simulink model "sideslip_hold"  (R2017a)
settings: Solver=FixedStepAuto  StartTime=0.0  StopTime=10  FixedStep=.001  RelTol=1e-3
values from neighbouring files (symbols this model uses):
  a_beta1 = -P.rho*Va*P.S_wing/(2*P.mass)*P.C_Y_beta    [computeRollGains.m]    (also in compute_gains.m)
  a_beta2 = P.rho*Va*P.S_wing/(2*P.mass)*P.C_Y_delta_r    [computeRollGains.m]    (also in compute_gains.m)
  delta_r_max = 45*pi/180    (= 0.785398163397)    [computeRollGains.m]    (also in compute_gains.m)
  ki_beta = 1/a_beta2*((a_beta1 + a_beta2*kp_beta)/2/zeta_beta)^2    [computeRollGains.m]
  kp_beta = delta_r_max/e_beta_max*sign(a_beta2)    [computeRollGains.m]
settings Model: Creator=pizzaslayer  LastModifiedBy=pizzaslayer

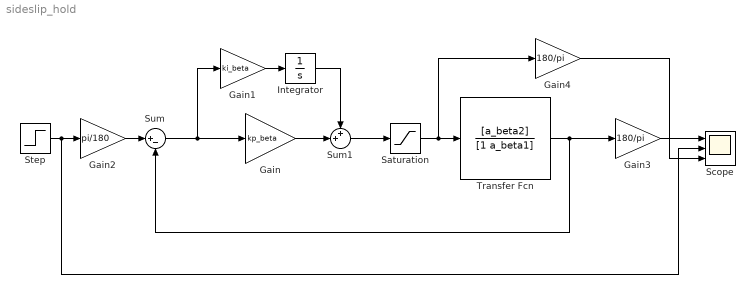
== system sideslip_hold ==
  Gain : Gain  Gain=kp_beta
  Gain1 : Gain  Gain=ki_beta
  Gain2 : Gain  Gain=pi/180
  Gain3 : Gain  Gain=180/pi
  Gain4 : Gain  Gain=180/pi
  Integrator : Integrator  InitialCondition=10*pi/180
  Saturation : Saturate  UpperLimit=delta_r_max  LowerLimit=-delta_r_max
  Scope : Scope  NumInputPorts=3
  Step : Step  Time=2  After=0  SampleTime=0
  Sum : Sum  Inputs=|+-
  Sum1 : Sum  Inputs=++|
  Transfer Fcn : TransferFcn  Numerator=[a_beta2]  Denominator=[1 a_beta1]
  wires:
  Step/1 -> Scope/2, Gain2/1
  Gain2/1 -> Sum/1
  Sum/1 -> Gain1/1, Gain/1
  Gain/1 -> Sum1/2
  Saturation/1 -> Gain4/1, Transfer Fcn/1
  Sum1/1 -> Saturation/1
  Transfer Fcn/1 -> Sum/2, Gain3/1
  Gain3/1 -> Scope/1
  Gain1/1 -> Integrator/1
  Integrator/1 -> Sum1/1
  Gain4/1 -> Scope/3
